simulink model "prob3"  (R2020a)
settings: Solver=VariableStepAuto  StartTime=0.0  StopTime=200  RelTol=1e-3
values from neighbouring files (symbols this model uses):
  c = 90.0    [datadic.sldd]    (also in para3.m = 90)
  c1 = 500.0    [datadic.sldd]    (also in para3.m = 500)
  ct = 10.0    [datadic.sldd]    (also in para3.m = 10)
  k = 100.0    [datadic.sldd]    (also in para3.m = 100)
  k1 = 100.0    [datadic.sldd]    (also in para3.m = 100)
  kt = 400.0    [datadic.sldd]    (also in para3.m = 400)
  m = 1000.0    [datadic.sldd]    (also in para3.m = 1000)
  m1 = 850.0    [datadic.sldd]    (also in para3.m = 850)
  m2 = 150.0    [datadic.sldd]    (also in para3.m = 150)
settings Model: DataDictionary=datadic.sldd  Creator=vijay  LastModifiedBy=vijay

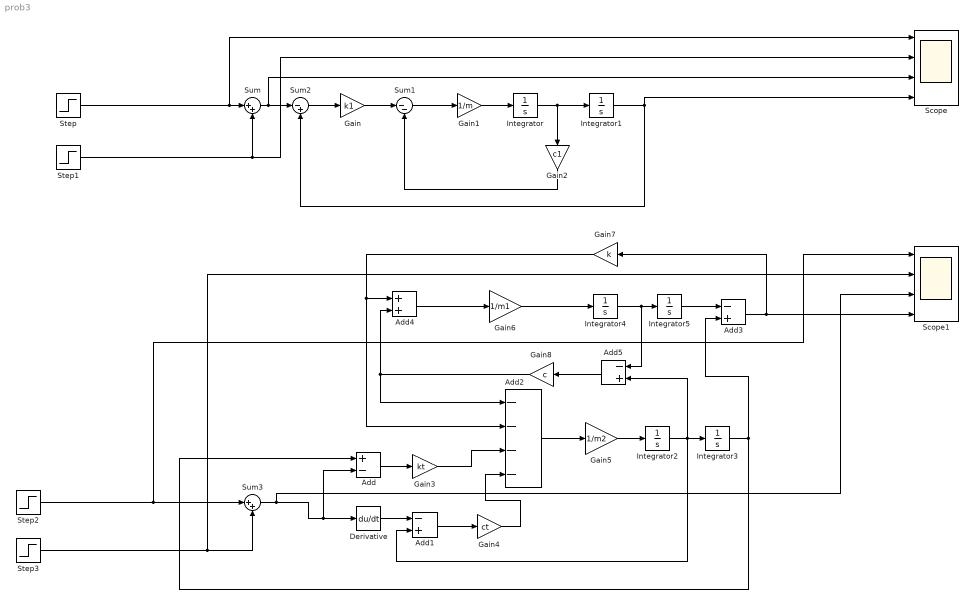
== system prob3 ==
  Add : Sum  Inputs=+-
  Add1 : Sum  Inputs=-+
  Add2 : Sum  Inputs=----
  Add3 : Sum  Inputs=-+
  Add4 : Sum
  Add5 : Sum  Inputs=-+
  Derivative : Derivative
  Gain : Gain  Gain=k1
  Gain1 : Gain  Gain=1/m
  Gain2 : Gain  Gain=c1
  Gain3 : Gain  Gain=kt
  Gain4 : Gain  Gain=ct
  Gain5 : Gain  Gain=1/m2
  Gain6 : Gain  Gain=1/m1
  Gain7 : Gain  Gain=k
  Gain8 : Gain  Gain=c
  Integrator{,1..5} (6 alike) : Integrator
  Scope : Scope  NumInputPorts=4
  Scope1 : Scope  NumInputPorts=4
  Step : Step  Before=15  After=0  SampleTime=45
  Step1 : Step  After=15  SampleTime=145
  Step2 : Step  Before=15  After=0  SampleTime=45
  Step3 : Step  After=15  SampleTime=145
  Sum : Sum  Inputs=|++
  Sum1 : Sum  Inputs=|--
  Sum2 : Sum  Inputs=|-+
  Sum3 : Sum  Inputs=|++
  wires:
  Sum/1 -> Scope/3, Sum2/1
  Sum2/1 -> Gain/1
  Gain/1 -> Sum1/1
  Sum1/1 -> Gain1/1
  Gain1/1 -> Integrator/1
  Integrator/1 -> Gain2/1, Integrator1/1
  Integrator1/1 -> Sum2/2, Scope/4
  Step/1 -> Scope/1, Sum/1
  Step1/1 -> Scope/2, Sum/2
  Gain2/1 -> Sum1/2
  Sum3/1 -> Scope1/3, Add/2, Derivative/1
  Step3/1 -> Scope1/2, Sum3/2
  Step2/1 -> Scope1/1, Sum3/1
  Integrator4/1 -> Add5/1, Integrator5/1
  Integrator2/1 -> Add1/2, Add5/2, Integrator3/1
  Integrator5/1 -> Add3/1
  Add3/1 -> Scope1/4, Gain7/1
  Derivative/1 -> Add1/1
  Add1/1 -> Gain4/1
  Gain4/1 -> Add2/4
  Integrator3/1 -> Add/1, Add3/2
  Gain6/1 -> Integrator4/1
  Add4/1 -> Gain6/1
  Gain7/1 -> Add2/2, Add4/1
  Gain8/1 -> Add2/1, Add4/2
  Add5/1 -> Gain8/1
  Gain5/1 -> Integrator2/1
  Add2/1 -> Gain5/1
  Add/1 -> Gain3/1
  Gain3/1 -> Add2/3
